simulink model "w3prob3"  (R2020a)
settings: Solver=VariableStepAuto  StartTime=0.0  StopTime=10.0  RelTol=1e-3
PostLoadFcn:
  | EMAP = [-40 -44 -49 -53 -57 -61 -65 -70 -74 -78 -82;215 117 85 66 44 29 10 -2 -13 -22 -32;245 208 178 148 122 104 85 66 48 33 18;264 260 241 219 193 167 152 133 119 96 85;264 279 282 275 260 238 223 208 189 171 152;267 290 293 297 290 275 260 256 234 212 193;267 297 305 305 305 301 293 282 267 249 226;267 301 308 312 319 323 319 316 297 279 253;267 301 312 319 327 327 327 327 312 293 267;267 301 312 319 327 334 334 334 319 305 275];
  | Iei = 0.0219914882835559;
  | TH_VEC = [0;20;30;40;50;60;70;80;90;100];
  | NE_VEC = [799.9999999999999 1200 1600 2000 2400 2800 3200 3600 4000 4400 4800];
  | CONVERTER_DATA = [0 137.4652089938063 2.232;0.1 137.065019156852 2.075;0.2 135.8644496459891 1.975;0.3 135.6643547275119 1.846;0.4 137.5652564530449 1.72;0.5 140.3665853117251 1.564;0.6 145.2689108144154 1.409;0.7 152.8725177165473 1.254;0.8 162.9773110996437 1.096;0.81 164.2779280697452 1.08;0.82 166.1788297952782 1.061;0.83 167.9796840615726 1.043;0.84 170.0806807055828 1.028;0.85 172.7819621050244 1.012;0.86 175.3831960452274 1.002;0.87 179.5851893332477 1.002;0.88 183.5870877027908 1.001;0.89 189.8900776348212 0.998;0.9 197.6937794554303 0.999;0.92 215.9024170368515 1.001;0.94 244.5159903790849 1.002];
  | UP_TABLE = [10 30 50 1000000;10 30 50 1000000;15 30 50 1000000;23 41 60 1000000;40 70 100 1000000;40 70 100 1000000];
  | UP_TH_BP = [0;25;35;50;90;100];
  | DOWN_TABLE = [0 5 20 35;0 5 20 35;0 5 25 40;0 5 30 50;0 30 50 80;0 30 50 80];
  | DOWN_TH_BP = [0;5;40;50;90;100];
  | TWAIT = 2;
model workspace (MAT data in the model file):
  CONVERTER_DATA = [0  137.465208994  2.232; 0.1  137.065019157  2.075; 0.2  135.864449646  1.975; 0.3  135.664354728  1.846; 0.4  137.565256453  1.72; 0.5  140.366585312  1.564; 0.6  145.268910814  1.409; 0.7  152.872517717  1.254; 0.8  162.9773111  1.096; 0.81  164.27792807  1.08; 0.82  166.178829795  1.061; 0.83  167.979684062  1.043; 0.84  170.080680706  1.028; 0.85  172.781962105  1.012; 0.86  175.383196045  1.002; 0.87  179.585189333  1.002; 0.88  183.587087703  1.001; 0.89  189.890077635  0.998; 0.9  197.693779455  0.999; 0.92  215.902417037  1.001; 0.94  244.515990379  1.002]
  Kfactor = [137.465208994; 137.065019157; 135.864449646; 135.664354728; 137.565256453; 140.366585312; 145.268910814; 152.872517717; 162.9773111; 164.27792807; 166.178829795; 167.979684062; 170.080680706; 172.781962105; 175.383196045; 179.585189333; 183.587087703; 189.890077635; 197.693779455; 215.902417037; 244.515990379]
  Torkratio = [2.232; 2.075; 1.975; 1.846; 1.72; 1.564; 1.409; 1.254; 1.096; 1.08; 1.061; 1.043; 1.028; 1.012; 1.002; 1.002; 1.001; 0.998; 0.999; 1.001; 1.002]
  speedratio = [0; 0.1; 0.2; 0.3; 0.4; 0.5; 0.6; 0.7; 0.8; 0.81; 0.82; 0.83; 0.84; 0.85; 0.86; 0.87; 0.88; 0.89; 0.9; 0.92; 0.94]
settings Model: Creator=Anjali123  LastModifiedBy=Anjali123

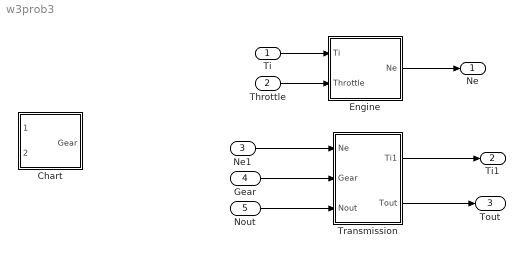
== system w3prob3 ==
  Ti : Inport  Unit=ft*lbf@torque
  Throttle : Inport  Port=2  Unit=%
  Ne1 : Inport  Port=3
  Gear : Inport  Port=4  Unit=1
  Nout : Inport  Port=5  Unit=rpm
  Chart : Stateflow chart  TreatAsAtomicUnit=on
  Engine : Subsystem
  Transmission : Subsystem
  Ne : Outport  Unit=rpm  VectorParamsAs1DForOutWhenUnconnected=off
  Ti1 : Outport  Port=2  VectorParamsAs1DForOutWhenUnconnected=off
  Tout : Outport  Port=3  Unit=ft*lbf@torque  VectorParamsAs1DForOutWhenUnconnected=off
  wires:
  Ti/1 -> Engine/1(Ti)
  Throttle/1 -> Engine/2(Throttle)
  Engine/1(Ne) -> Ne/1
  Ne1/1 -> Transmission/1(Ne)
  Gear/1 -> Transmission/2(Gear)
  Nout/1 -> Transmission/3(Nout)
  Transmission/1(Ti1) -> Ti1/1
  Transmission/2(Tout) -> Tout/1

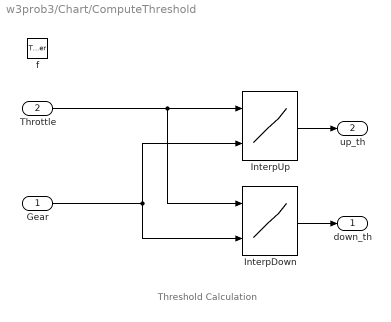
== system w3prob3/Chart/ComputeThreshold ==
  note: Threshold Calculation
  Gear : Inport
  Throttle : Inport  Port=2
  f : TriggerPort  TriggerType=function-call  VariantControl=(inherit)
      settings: CopyFcn=Stateflow.SLINSF.SimulinkMan.removeBlockPreDeleteFcn  PreDeleteFcn=Stateflow.SLINSF.SimulinkMan.unsafePredeleteFcn
  InterpDown : Lookup_n-D  BreakpointsForDimension1=DOWN_TH_BP  BreakpointsForDimension2=[1:4]  Table=DOWN_TABLE  OutDataTypeStr=double  LockScale=on
  InterpUp : Lookup_n-D  BreakpointsForDimension1=UP_TH_BP  BreakpointsForDimension2=[1:4]  Table=UP_TABLE  OutDataTypeStr=double  LockScale=on
  down_th : Outport  InitialOutput=0  VectorParamsAs1DForOutWhenUnconnected=off
  up_th : Outport  Port=2  InitialOutput=0  VectorParamsAs1DForOutWhenUnconnected=off
  wires:
  InterpUp/1 -> up_th/1
  InterpDown/1 -> down_th/1
  Throttle/1 -> InterpDown/1, InterpUp/1
  Gear/1 -> InterpDown/2, InterpUp/2

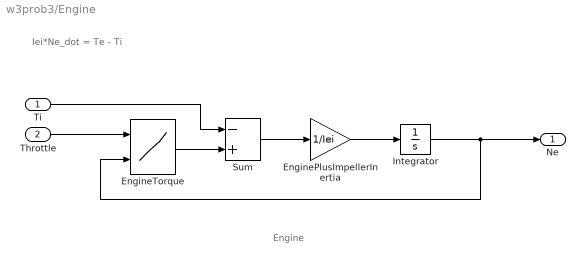
== system w3prob3/Engine ==
  note: Engine
  note: Iei*Ne_dot = Te - Ti
  Ti : Inport  Unit=ft*lbf@torque
  Throttle : Inport  Port=2  Unit=%
  EnginePlusImpellerInertia : Gain  Gain=1/Iei  SaturateOnIntegerOverflow=on  OutDataTypeStr=Inherit: Same as input  ParamDataTypeStr=Inherit: Same as input
  EngineTorque : Lookup_n-D  BreakpointsForDimension1=TH_VEC  BreakpointsForDimension2=NE_VEC  Table=EMAP  InputSameDT=on
  Integrator : Integrator  InitialCondition=1000  LimitOutput=on  UpperSaturationLimit=6000  LowerSaturationLimit=600  ZeroCross=off
  Sum : Sum  Inputs=-+  InputSameDT=on  SaturateOnIntegerOverflow=on  OutDataTypeStr=Inherit: Same as first input
  Ne : Outport  Unit=rpm  VectorParamsAs1DForOutWhenUnconnected=off
  wires:
  EngineTorque/1 -> Sum/2
  EnginePlusImpellerInertia/1 -> Integrator/1
  Integrator/1 -> Ne/1, EngineTorque/2
  Sum/1 -> EnginePlusImpellerInertia/1
  Throttle/1 -> EngineTorque/1
  Ti/1 -> Sum/1

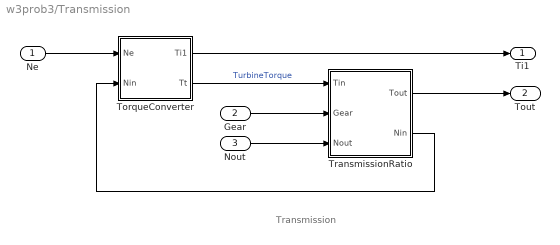
== system w3prob3/Transmission ==
  note: Transmission
  Ne : Inport
  Gear : Inport  Port=2  Unit=1
  Nout : Inport  Port=3  Unit=rpm
  TorqueConverter : Subsystem
  TransmissionRatio : Subsystem
  Ti1 : Outport  VectorParamsAs1DForOutWhenUnconnected=off
  Tout : Outport  Port=2  Unit=ft*lbf@torque  VectorParamsAs1DForOutWhenUnconnected=off
  wires:
  Ne/1 -> TorqueConverter/1(Ne)
  TorqueConverter/2(Tt) -> TransmissionRatio/1(Tin)  "TurbineTorque"
  TransmissionRatio/1(Tout) -> Tout/1
  Gear/1 -> TransmissionRatio/2(Gear)
  TransmissionRatio/2(Nin) -> TorqueConverter/2(Nin)
  TorqueConverter/1(Ti1) -> Ti1/1
  Nout/1 -> TransmissionRatio/3(Nout)

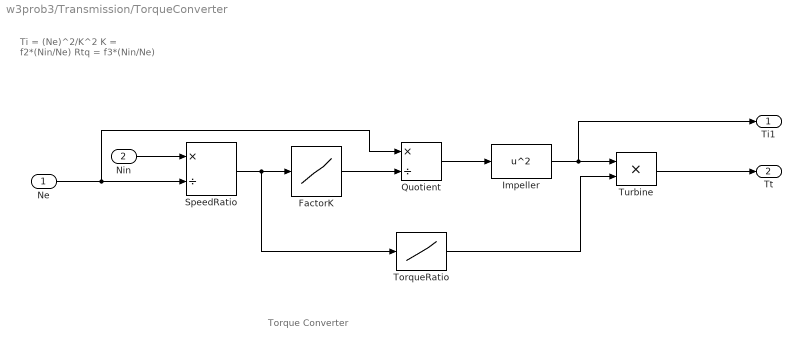
== system w3prob3/Transmission/TorqueConverter ==
  note: Ti = (Ne)^2/K^2
      | K = f2*(Nin/Ne)
      | Rtq = f3*(Nin/Ne)
  note: Torque Converter
  Ne : Inport
  Nin : Inport  Port=2
  FactorK : Lookup_n-D  NumberOfTableDimensions=1  BreakpointsForDimension1=speedratio  Table=Kfactor  SaturateOnIntegerOverflow=on  InputSameDT=on
  Impeller : Fcn  Expr=u^2
  Quotient : Product  Inputs=*/  InputSameDT=on  SaturateOnIntegerOverflow=on  OutDataTypeStr=Inherit: Same as first input
  SpeedRatio : Product  Inputs=*/  InputSameDT=on  SaturateOnIntegerOverflow=on  OutDataTypeStr=Inherit: Same as first input
  TorqueRatio : Lookup_n-D  NumberOfTableDimensions=1  BreakpointsForDimension1=speedratio  Table=Torkratio  SaturateOnIntegerOverflow=on  InputSameDT=on
  Turbine : Product  InputSameDT=on  SaturateOnIntegerOverflow=on  OutDataTypeStr=Inherit: Same as first input
  Ti1 : Outport  VectorParamsAs1DForOutWhenUnconnected=off
  Tt : Outport  Port=2  VectorParamsAs1DForOutWhenUnconnected=off
  wires:
  TorqueRatio/1 -> Turbine/2
  Turbine/1 -> Tt/1
  Ne/1 -> Quotient/1, SpeedRatio/2
  Impeller/1 -> Ti1/1, Turbine/1
  Nin/1 -> SpeedRatio/1
  SpeedRatio/1 -> FactorK/1, TorqueRatio/1
  FactorK/1 -> Quotient/2
  Quotient/1 -> Impeller/1

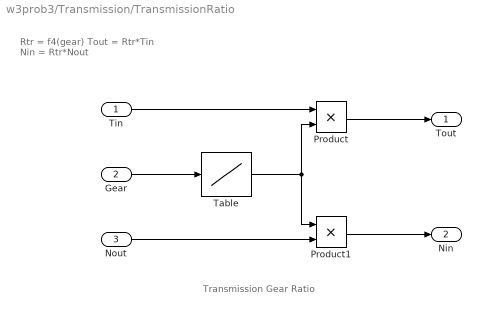
== system w3prob3/Transmission/TransmissionRatio ==
  note: Rtr = f4(gear)
      | Tout = Rtr*Tin
      | Nin = Rtr*Nout
  note: Transmission Gear Ratio
  Tin : Inport  Unit=ft*lbf@torque
  Gear : Inport  Port=2  Unit=1
  Nout : Inport  Port=3  Unit=rpm
  Product : Product  InputSameDT=on  SaturateOnIntegerOverflow=on  OutDataTypeStr=Inherit: Same as first input
  Product1 : Product  InputSameDT=on  SaturateOnIntegerOverflow=on  OutDataTypeStr=Inherit: Same as first input
  Table : Lookup_n-D  NumberOfTableDimensions=1  BreakpointsForDimension1=[1 2 3 4]  Table=[2.393 1.450 1.000 0.677]  OutDataTypeStr=double  SaturateOnIntegerOverflow=on  InputSameDT=on  LockScale=on
  Tout : Outport  Unit=ft*lbf@torque  VectorParamsAs1DForOutWhenUnconnected=off
  Nin : Outport  Port=2  Unit=rpm  VectorParamsAs1DForOutWhenUnconnected=off
  wires:
  Table/1 -> Product1/1, Product/2
  Product/1 -> Tout/1
  Nout/1 -> Product1/2
  Tin/1 -> Product/1
  Product1/1 -> Nin/1
  Gear/1 -> Table/1

== stateflow chart w3prob3/Chart ==
  state gear_state [parallel]
    settings: executionOrder=1
    state first
      entry:
      Gear = 1;
    state second
      entry:
      Gear = 2;
    state third
      entry:
      Gear = 3;
    state fourth
      entry:
      Gear = 4;
    (default) -> first
    second -> third [order 1] : UP
    first -> second : UP
    third -> fourth [order 1] : UP
    third -> second [order 2] : DOWN
    second -> first [order 2] : DOWN
    fourth -> third : DOWN
  state selection_state [parallel]
    during:
    [down_th, up_th] = ComputeThreshold(Gear,Throttle);
    settings: executionOrder=2
    state steady_state
    state upshifting
    state downshifting
    (default) -> steady_state
    steady_state -> upshifting [order 1] : [VehicleSpeed > up_th]
    steady_state -> downshifting [order 2] : [VehicleSpeed < down_th]
    downshifting -> steady_state [order 1] : after(TWAIT,tick)
        | [VehicleSpeed <= down_th]
        | {gear_state.DOWN}
    downshifting -> steady_state [order 2] : [VehicleSpeed > down_th]
    upshifting -> steady_state [order 1] : after(TWAIT,tick)
        | [VehicleSpeed >= up_th]
        | {gear_state.UP}
    upshifting -> steady_state [order 2] : [VehicleSpeed < up_th]
  state [down_th,up_th] = ComputeThreshold(Gear,Throttle) [function]
  data: Gear function_input; Throttle function_input; down_th function_output; up_th function_output; Throttle input; VehicleSpeed input; down_th local; up_th local; TWAIT parameter; Gear output
  events: DOWN local EITHER_EDGE_EVENT; UP local EITHER_EDGE_EVENT
